simulink model "Forward_Converter_controller"  (R2018a)
settings: Solver=VariableStepAuto  StartTime=0.0  StopTime=0.01  MaxStep=1e-4  RelTol=1e-4  EnableMultiTasking=on
undefined symbols (not defined in the file): sigbuilder_block
libraries: powerlib x22, simulink x2
Description:
  | Copyright 2008-2018 The MathWorks, Inc.
settings Model: Creator=MathWorks  LastModifiedBy=Ekin Su Saçın
settings SolverCC: SolverResetMethod=Robust
settings DataIOCC: ReturnWorkspaceOutputs=on
settings OptimizationCC: LifeSpan=inf
settings DebuggingCC: ReadBeforeWriteMsg=DisableAll  WriteAfterWriteMsg=DisableAll  WriteAfterReadMsg=DisableAll  MultiTaskDSMMsg=none  SFUnexpectedBacktrackingDiag=warning  SFNoUnconditionalDefaultTransitionDiag=warning  SFExecutionAtInitializationDiag=none
settings ModelReferenceCC: UpdateModelReferenceTargets=IfOutOfDate
settings SFSimCC: SFSimEcho=off
settings CodeAppCC: StateflowObjectComments=on
settings GRTTargetCC: TargetLangStandard=C89/C90 (ANSI)  GeneratePreprocessorConditionals=Disable all
settings ConfigComp: CovMetricSettings=dw  CovHtmlReporting=on  CovSaveCumulativeToWorkspaceVar=on  CovSaveSingleToWorkspaceVar=on  CovExternalEMLEnable=off
settings SimscapeCC: SimscapeNormalizeSystem=off  SimscapeNominalValues={1, 'bar'; 1, 'cm^3/s'; 1, 'bar*kg/s'; 1, 'kJ/kg'; 1, 'kW'; }

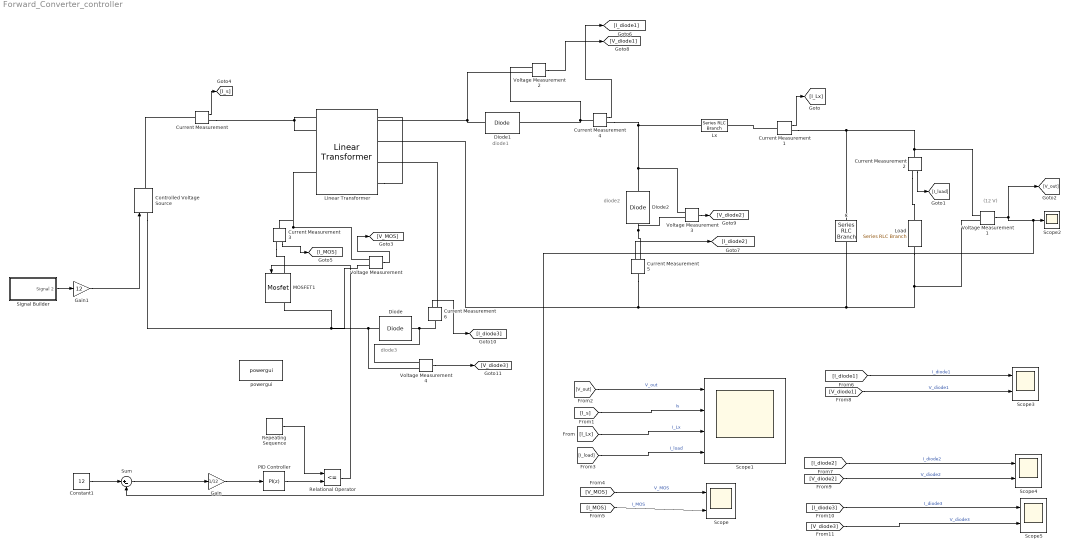
== system Forward_Converter_controller ==
  note: diode1
  note: (12 V)
  note: diode2
  note: diode3
  C : powerlib/Elements/Series RLC Branch  LConnTagsString=__new0  RConnTagsString=__new0  BranchType=C  Resistance=1e-4  Inductance=200e-6  SetiL0=off  InitialCurrent=0  Capacitance=100e-6  Setx0=off  InitialVoltage=0  Measurements=None
  Constant1 : Constant  Value=12
  Controlled Voltage Source : powerlib/Electrical Sources/Controlled Voltage Source  Initialize=on  Source_Type=AC  Amplitude=0  Phase=0  Frequency=0  Measurements=None
  Current Measurement{,1..6} (7 alike) : powerlib/Measurements/Current Measurement  PhasorSimulation=off  OutputType=Complex  PSBequivalent=0
  Diode : powerlib/Power Electronics/Diode  Ron=0.001  Lon=0  Vf=1.2  IC=0  UseSnubber=0  Rs=500  Cs=250e-9  Measurements=off
  Diode1 : powerlib/Power Electronics/Diode  Ron=17.7e-3  Lon=0  Vf=0.85  IC=0  UseSnubber=0  Rs=500  Cs=250e-9  Measurements=off
  Diode2 : powerlib/Power Electronics/Diode  Ron=0.001  Lon=0  Vf=0.85  IC=0  UseSnubber=0  Rs=500  Cs=250e-9  Measurements=off
  Gain : Gain  Gain=1/12
  Gain1 : Gain  Gain=12
  Linear Transformer : powerlib/Elements/Linear Transformer  UNITS=SI  NominalPower=[ 25 35e3 ]  winding1=[15 0.0219 1e-06]  winding2=[20 0.0331 1e-06]  ThreeWindings=on  winding3=[15 5e-03 1e-06]  RmLm=[500 0.66e-3]  Measurements=Magnetization current  DataType=on
  Load : powerlib/Elements/Series RLC Branch  LConnTagsString=__new0  RConnTagsString=__new0  BranchType=R  Resistance=2.87  Inductance=200e-6  SetiL0=off  InitialCurrent=0  Capacitance=400e-6  Setx0=off  InitialVoltage=0  Measurements=Branch current
  Lx : powerlib/Elements/Series RLC Branch  LConnTagsString=__new0  RConnTagsString=__new0  BranchType=L  Resistance=10  Inductance=400e-6  SetiL0=off  InitialCurrent=0  Capacitance=400e-6  Setx0=off  InitialVoltage=0  Measurements=Branch current
  MOSFET1 : powerlib/Power Electronics/Mosfet  Ron=77e-3  Lon=0  Rd=1e-3  Vfd=1  IC=0  Rs=1e6  Cs=inf  Measurements=on
  PID Controller : simulink/Continuous/PID Controller  Controller=PI  TimeDomain=Discrete-time  SampleTime=-1  IntegratorMethod=Forward Euler  FilterMethod=Forward Euler  Form=Parallel  UseFilter=on  ControllerParametersSource=internal  P=.7  I=100  D=0  N=100  InitialConditionSource=internal  InitialConditionForIntegrator=0  InitialConditionForFilter=0  ExternalReset=none  LimitOutput=on  UpperSaturationLimit=.9  LowerSaturationLimit=.1  LinearizeAsGain=on  AntiWindupMode=none  Kb=1  TrackingMode=off  Kt=1  PParamMin=[]  PParamMax=[]  IParamMin=[]  IParamMax=[]  DParamMin=[]  DParamMax=[]  NParamMin=[]  NParamMax=[]  KbParamMin=[]  KbParamMax=[]  KtParamMin=[]  KtParamMax=[]  POutMin=[]  POutMax=[]  IOutMin=[]  IOutMax=[]  DOutMin=[]  DOutMax=[]  NOutMin=[]  NOutMax=[]  KbOutMin=[]  KbOutMax=[]  KtOutMin=[]  KtOutMax=[]  IntegratorOutMin=[]  IntegratorOutMax=[]  FilterOutMin=[]  FilterOutMax=[]  SumOutMin=[]  SumOutMax=[]  SumI1OutMin=[]  SumI1OutMax=[]  SumI2OutMin=[]  SumI2OutMax=[]  SumI3OutMin=[]  SumI3OutMax=[]  SumDOutMin=[]  SumDOutMax=[]  SaturationOutMin=[]  SaturationOutMax=[]  IntegratorContinuousStateAttributes=''  IntegratorStateMustResolveToSignalObject=off  IntegratorRTWStateStorageClass=Auto  FilterContinuousStateAttributes=''  FilterStateMustResolveToSignalObject=off  FilterRTWStateStorageClass=Auto  DifferentiatorICPrevScaledInput=0  DifferentiatorOutMin=[]  DifferentiatorOutMax=[]  FilterDiffOutCoefMin=[]  FilterDiffOutCoefMax=[]  SumDenOutMin=[]  SumDenOutMax=[]  SumNumOutMin=[]  SumNumOutMax=[]  ReciprocalOutMin=[]  ReciprocalOutMax=[]  DivideOutMin=[]  DivideOutMax=[]  TunerSelectOption=Transfer Function Based (PID Tuner App)
  Relational Operator : RelationalOperator  Operator=<=  OutDataTypeStr=boolean  RndMeth=Simplest
  Repeating Sequence : simulink/Sources/Repeating Sequence  rep_seq_t=[0 .00004]  rep_seq_y=[0 1]
  Scope{,3..5} (4 alike) : Scope  NumInputPorts=2
  Scope1 : Scope  NumInputPorts=4
  Scope2 : Scope
  Signal Builder : Subsystem  Tag=STV Subsys  LoadFcn=sigbuilder_block('load');  StartFcn=sigbuilder_block('start');  StopFcn=sigbuilder_block('stop');  ClipboardFcn=sigbuilder_block('clipboard');  mask(Sigbuilder block){tuvar=[0:10]}
      mask help: Simulink:masks:SigbuilderBlock_MD
      mask init:
      | if ~strcmp(get_param(bdroot(gcbh),'SimulationStatus'),'stopped') tuvar = sigbuilder_block('maskInit'); end
      settings: CopyFcn=sigbuilder_block('copy');  DeleteFcn=sigbuilder_block('delete');  ModelCloseFcn=sigbuilder_block('modelClose');  PreSaveFcn=sigbuilder_block('preSave');  PauseFcn=sigbuilder_block('pause');  ContinueFcn=sigbuilder_block('continue');  NameChangeFcn=sigbuilder_block('namechange');  OpenFcn=sigbuilder_block('open',[437.6 199.2 550.4 400 ]);  CloseFcn=sigbuilder_block('close');
      mask Display: plot(0, 0, 100, 100,[2, 2, 32, 32, 2], [68, 8, 8, 68, 68],[32, 2], [38, 38], [32, 19, 2],[53, 60, 44], [32, 17, 17, 2],[16, 16, 31, 31]);txt = getActiveGroup(gcbh);text(2, 100, txt,'verticalAlignment', 'top');
  Sum : Sum  Inputs=|+-
  Voltage Measurement{,1..4} (5 alike) : powerlib/Measurements/Voltage Measurement  PhasorSimulation=off  OutputType=Complex  PSBequivalent=0
  powergui : powerlib/powergui  Priority=1  SimulationMode=Continuous  SampleTime=50e-6  frequency=60  Iterations=50  frequencyindice=0  Pbase=100e6  ErrMax=1e-4  UnitsV=kV  UnitsW=MW  buscounter=0  FunctionMessages=off  echomessages=off  EnableUseOfTLC=off  CurrentSourceSwitches=off  DisableSnubberDevices=off  DisableRonSwitches=off  DisableVfSwitches=off  DisplayEquations=off  SolverType=Tustin/Backward Euler (TBE)  Interpol=off  ExternalGateDelay=off  methode=off  Ts=100  x0status=blocks  SPID=on  SwTol=0  HookPort=off  RestoreLinks=warning  ResistiveCurrentMeasurement=off  Frange=[0:2:500]  Ylog=off  Xlog=on  ShowGrid=off  save=off  variable=ZData  structure=0  ZoomFFT=off  StartTime=0.0  cycles=1  DisplayStyle=1  fundamental=60  FreqAxis=off  MaxFrequency=1000  frequencyindicesteady=1  RmsSteady=1  display=off
  wires:
  Voltage Measurement1/1 -> [V_out], Sum/2, Scope2/1
  Current Measurement/1 -> [I_s]
  [I_s] -> Scope1/2  "Is"
  Current Measurement1/1 -> [I_Lx]
  Current Measurement2/1 -> [I_load]
  [I_Lx] -> Scope1/3  "I_Lx"
  [I_load] -> Scope1/4  "I_load"
  [V_out] -> Scope1/1  "V_out"
  Voltage Measurement/1 -> [V_MOS]
  [V_MOS] -> Scope/1  "V_MOS"
  Current Measurement3/1 -> [I_MOS]
  [I_MOS] -> Scope/2  "I_MOS"
  Current Measurement4/1 -> [I_diode1]
  [I_diode1] -> Scope3/1  "I_diode1"
  [V_diode1] -> Scope3/2  "V_diode1"
  [I_diode2] -> Scope4/1  "I_diode2"
  [V_diode2] -> Scope4/2  "V_diode2"
  Current Measurement5/1 -> [I_diode2]
  Voltage Measurement2/1 -> [V_diode1]
  Voltage Measurement3/1 -> [V_diode2]
  Current Measurement6/1 -> [I_diode3]
  Voltage Measurement4/1 -> [V_diode3]
  [I_diode3] -> Scope5/1  "I_diode3"
  [V_diode3] -> Scope5/2  "V_diode3"
  Repeating Sequence/1 -> Relational Operator/1
  PID Controller/1 -> Relational Operator/2
  Gain/1 -> PID Controller/1
  Relational Operator/1 -> MOSFET1/1
  Constant1/1 -> Sum/1
  Sum/1 -> Gain/1
  Gain1/1 -> Controlled Voltage Source/1
  Signal Builder/1(Signal 2) -> Gain1/1
  connections:
  Current Measurement1/RConn1 -- Voltage Measurement1/LConn1 -- Current Measurement2/LConn1 -- C/LConn1
  Load/RConn1 -- Voltage Measurement1/LConn2 -- Linear Transformer/RConn2 -- Current Measurement5/LConn1 -- C/RConn1
  Voltage Measurement/LConn1 -- Current Measurement3/LConn1 -- Linear Transformer/LConn2
  MOSFET1/RConn1 -- Controlled Voltage Source/LConn1 -- Voltage Measurement4/LConn2 -- Diode/LConn1 -- Voltage Measurement/LConn2
  Linear Transformer/RConn4 -- Current Measurement/RConn1 -- Linear Transformer/LConn1
  Diode1/LConn1 -- Voltage Measurement2/LConn2 -- Linear Transformer/RConn1
  Diode2/RConn1 -- Voltage Measurement3/LConn1 -- Current Measurement4/RConn1 -- Lx/LConn1
  Controlled Voltage Source/RConn1 -- Current Measurement/LConn1
  Current Measurement1/LConn1 -- Lx/RConn1
  Current Measurement2/RConn1 -- Load/LConn1
  Current Measurement3/RConn1 -- MOSFET1/LConn1
  Current Measurement4/LConn1 -- Voltage Measurement2/LConn1 -- Diode1/RConn1
  Current Measurement5/RConn1 -- Voltage Measurement3/LConn2 -- Diode2/LConn1
  Diode/RConn1 -- Voltage Measurement4/LConn1 -- Current Measurement6/LConn1
  Current Measurement6/RConn1 -- Linear Transformer/RConn3

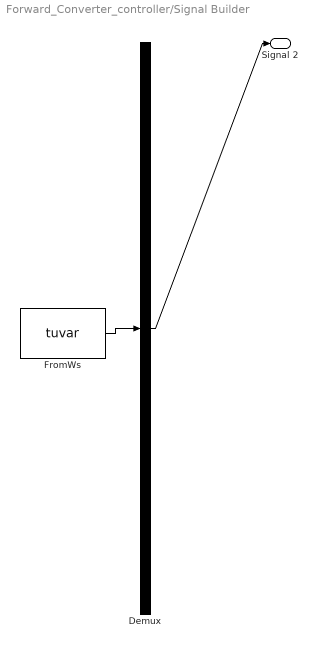
== system Forward_Converter_controller/Signal Builder ==
  Demux : Demux  Tag=STV Demux  Outputs=1
  FromWs : FromWorkspace  Tag=STV FromWs  VariableName=tuvar  SampleTime=0
      SigBuilderData=|
      | common.afterFinalStr = 'Extrapolate'
      | common.sampleTime = 0
      | dataSet.timeRange = [0 4]
      | dataSet.name = 'Group 1'
      | sbobj.Groups.Name = 'Group 1'
      | sbobj.Groups.Signals.Name = 'Signal 2'
      | sbobj.Groups.Signals.XData = [0 1 1 2 2 3 3 4]
      | sbobj.Groups.Signals.YData = [0.6 0.6 0.7 0.7 0.75 0.75 0.65 0.65]
      | sbobj.Groups.TimeRange = [0 4]
  Signal 2 : Outport  Tag=STV Outport
  wires:
  FromWs/1 -> Demux/1
  Demux/1 -> Signal 2/1
